simulink model "CANTXcommunicationunit_1"  (R2024a)
settings: Solver=VariableStepAuto  StartTime=0.0  StopTime=10.0  RelTol=1e-3
undefined symbols (not defined in the file or in its folder): canChannel
libraries: canlib x4, canmsglib x3
settings Model: DataDictionary=BMS_System_dict1.sldd  Creator=hirah  LastModifiedBy=hirah

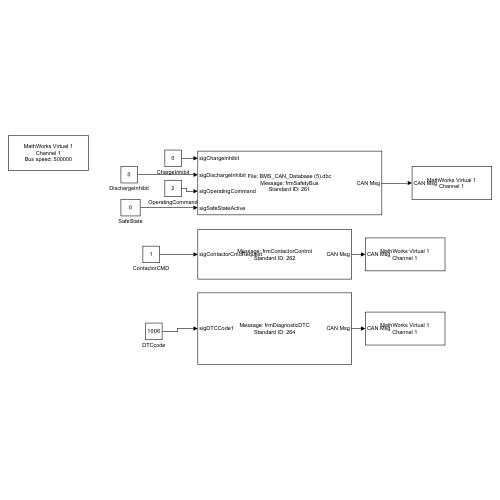
[thumbnail: Simulink's stored preview of the top-level diagram]
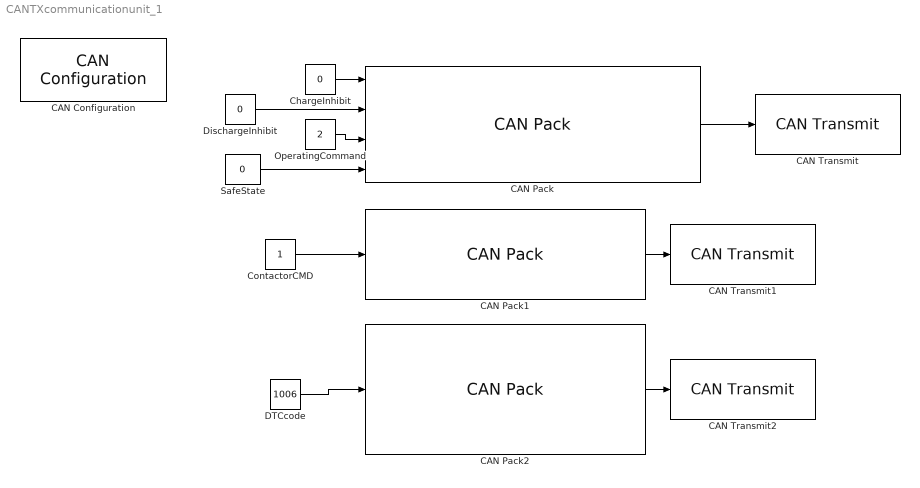
== system CANTXcommunicationunit_1 ==
  CAN Configuration : canlib/CAN Configuration  BlockHandle=406.0005  Device=MathWorks Virtual 1 (Channel 1)  DeviceMenu=MathWorks Virtual 1 (Channel 1)  ObjConstructor=canChannel('MathWorks', 'Virtual 1', 1)  BusSpeed=500000  EnableBitParameters=off  AckMode=Normal
  CAN Pack : canmsglib/CAN Pack  CANdbFile=C:\Users\hirah\Downloads\BMS_CAN_Database (5).dbc  MsgList=frmSafetyBus  MsgName=frmSafetyBus  MsgIDType=Standard (11-bit identifier)  MsgIdentifier=261  MsgLength=4  Remote=off  ApplyMinMax=off  BusOutput=off  SignalInfo={'sigChargeInhibit','8','8','LE','unsigned','Standard','0','1','0','0','1';'sigDischargeInhibit','16','8','LE','unsigned','Standard','0','1','0','0','1';'sigOperatingCommand','24','8','LE','unsigned','Standard','0','1','0','0','5';'sigSafeStateActive','0','8','LE','unsigned','Standard','0','1','0','0','1'}
      settings: LibrarySourceBlock=canlib/CAN Pack  DataFormat=CANdb specified signals
  CAN Pack1 : canmsglib/CAN Pack  CANdbFile=C:\Users\hirah\Downloads\BMS_CAN_Database (5).dbc  MsgList=frmContactorControl  MsgName=frmContactorControl  MsgIDType=Standard (11-bit identifier)  MsgIdentifier=262  MsgLength=3  Remote=off  ApplyMinMax=off  BusOutput=off  SignalInfo={ 'sigContactorCmdRequest', '0', '8', 'LE', 'unsigned', 'Standard', '0', '1', '0', '0', '7' }
      settings: LibrarySourceBlock=canlib/CAN Pack  DataFormat=manually specified signals
  CAN Pack2 : canmsglib/CAN Pack  CANdbFile=C:\Users\hirah\Downloads\BMS_CAN_Database (5).dbc  MsgList=frmDiagnosticDTC  MsgName=frmDiagnosticDTC  MsgIDType=Standard (11-bit identifier)  MsgIdentifier=264  MsgLength=3  Remote=off  ApplyMinMax=off  BusOutput=off  SignalInfo={ 'sigDTCCode1', '0', '16', 'LE', 'unsigned', 'Standard', '0', '1', '0', '0', '65535' }
      settings: LibrarySourceBlock=canlib/CAN Pack  DataFormat=manually specified signals
  CAN Transmit : canlib/CAN Transmit  BlockHandle=419.0002  Device=MathWorks Virtual 1 (Channel 1)  DeviceMenu=MathWorks Virtual 1 (Channel 1)  ObjConstructor=canChannel('MathWorks', 'Virtual 1', 1)  EnableEventTransmit=off  EnablePeriodicTransmit=off  MessagePeriod=1.000
  CAN Transmit1 : canlib/CAN Transmit  BlockHandle=421.0001  Device=MathWorks Virtual 1 (Channel 1)  DeviceMenu=MathWorks Virtual 1 (Channel 1)  ObjConstructor=canChannel('MathWorks', 'Virtual 1', 1)  EnableEventTransmit=off  EnablePeriodicTransmit=off  MessagePeriod=1.000
  CAN Transmit2 : canlib/CAN Transmit  BlockHandle=423.0001  Device=MathWorks Virtual 1 (Channel 1)  DeviceMenu=MathWorks Virtual 1 (Channel 1)  ObjConstructor=canChannel('MathWorks', 'Virtual 1', 1)  EnableEventTransmit=off  EnablePeriodicTransmit=off  MessagePeriod=1.000
  ChargeInhibit : Constant  Value=0  OutDataTypeStr=uint8
  ContactorCMD : Constant  OutDataTypeStr=uint8
  DTCcode : Constant  Value=1006
  DischargeInhibit : Constant  Value=0  OutDataTypeStr=uint8
  OperatingCommand : Constant  Value=2  OutDataTypeStr=uint8
  SafeState : Constant  Value=0  OutDataTypeStr=uint8
  wires:
  ChargeInhibit/1 -> CAN Pack/1
  DischargeInhibit/1 -> CAN Pack/2
  OperatingCommand/1 -> CAN Pack/3
  SafeState/1 -> CAN Pack/4
  CAN Pack/1 -> CAN Transmit/1
  ContactorCMD/1 -> CAN Pack1/1
  DTCcode/1 -> CAN Pack2/1
  CAN Pack2/1 -> CAN Transmit2/1
  CAN Pack1/1 -> CAN Transmit1/1
